simulink model "pendule"  (R2019a)
settings: Solver=VariableStepAuto  StartTime=0.0  StopTime=10.0  RelTol=1e-3
libraries: simulink x1
settings Model: Creator=nfoin  LastModifiedBy=nfoin

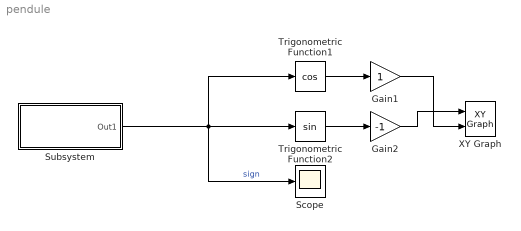
== system pendule ==
  Gain1 : Gain
  Gain2 : Gain  Gain=-1
  Scope : Scope
  Subsystem : Subsystem
  Trigonometric Function1 : Trigonometry  Operator=cos
  Trigonometric Function2 : Trigonometry
  XY Graph : simulink/Sinks/XY Graph  xmin=-10  xmax=10  ymin=-10  ymax=10  st=-1
  wires:
  Trigonometric Function1/1 -> Gain1/1
  Gain1/1 -> XY Graph/2
  Trigonometric Function2/1 -> Gain2/1
  Gain2/1 -> XY Graph/1
  Subsystem/1(Out1) -> Scope/1, Trigonometric Function2/1, Trigonometric Function1/1  "sign"

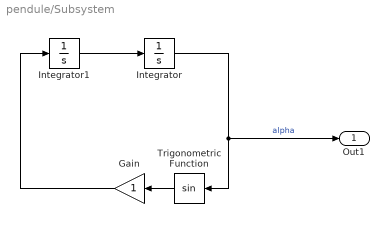
== system pendule/Subsystem ==
  Gain : Gain
  Integrator : Integrator
  Integrator1 : Integrator  InitialCondition=1
  Trigonometric Function : Trigonometry
  Out1 : Outport
  wires:
  Gain/1 -> Integrator1/1
  Trigonometric Function/1 -> Gain/1
  Integrator/1 -> Out1/1, Trigonometric Function/1  "alpha"
  Integrator1/1 -> Integrator/1
